simulink subsystem "VanDerPol"  (R2023a)
settings: Solver=VariableStepAuto  StartTime=0.0  StopTime=10.0  RelTol=1e-3
settings Model: Creator=KozlovM  LastModifiedBy=KozlovM

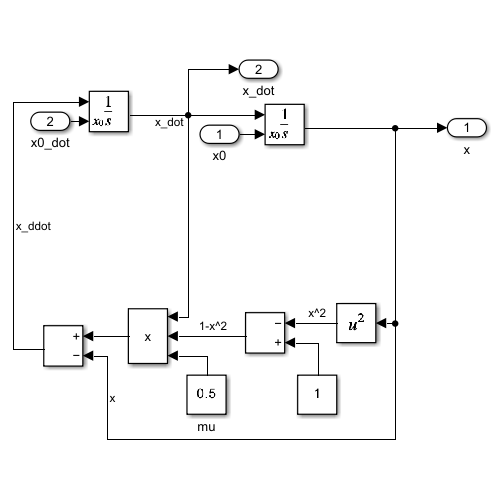
[thumbnail: Simulink's stored preview of the top-level diagram]
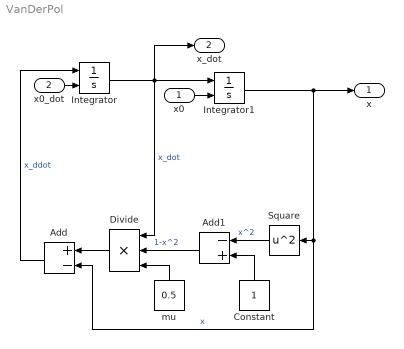
== system VanDerPol ==
  x0 : Inport
  x0_dot : Inport  Port=2
  Add : Sum  Inputs=+-
  Add1 : Sum  Inputs=-+
  Constant : Constant
  Divide : Product  Inputs=***
  Integrator : Integrator  InitialConditionSource=external
  Integrator1 : Integrator  InitialConditionSource=external  InitialCondition=2
  Square : Math  Operator=square
  mu : Constant  Value=0.5
  x : Outport
  x_dot : Outport  Port=2
  wires:
  Add1/1 -> Divide/2  "1-x^2"
  Constant/1 -> Add1/2
  mu/1 -> Divide/3
  Add/1 -> Integrator/1  "x_ddot"
  Integrator1/1 -> Add/2, Square/1, x/1  "x"
  Integrator/1 -> x_dot/1, Divide/1, Integrator1/1  "x_dot"
  Square/1 -> Add1/1  "x^2"
  Divide/1 -> Add/1
  x0_dot/1 -> Integrator/2
  x0/1 -> Integrator1/2
